simulink model "p4"  (R2020b)
settings: Solver=VariableStepAuto  StartTime=0.0  StopTime=10.0  RelTol=1e-3
model workspace (MAT data in the model file):
  a = 0.5
  b = 0.25
  x = 0.4
libraries: simulink x1
settings Model: OrderedModelArguments=off  Creator=DELL  LastModifiedBy=DELL

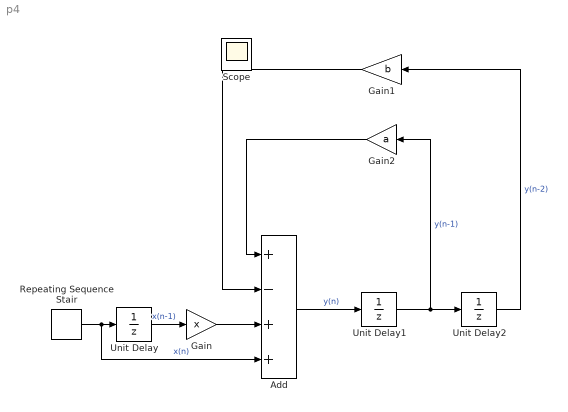
== system p4 ==
  Add : Sum  Inputs=+-++
  Gain : Gain  Gain=x
  Gain1 : Gain  Gain=b
  Gain2 : Gain  Gain=a
  Repeating Sequence Stair : simulink/Sources/Repeating Sequence Stair  OutValues=[3 1 4 2 1].'  tsamp=-1  OutMin=[]  OutMax=[]  OutDataTypeStr=double  OutputDataTypeScalingMode=double  OutDataType=fixdt(0,8)  ConRadixGroup=Best Precision: Vector-wise  OutScaling=2^-12
  Unit Delay : UnitDelay  SampleTime=-1  HasFrameUpgradeWarning=on
  Unit Delay1 : UnitDelay  SampleTime=-1  HasFrameUpgradeWarning=on
  Unit Delay2 : UnitDelay  SampleTime=-1  HasFrameUpgradeWarning=on
  Scope : Scope
  wires:
  Gain1/1 -> Add/2
  Add/1 -> Unit Delay1/1  "y(n)"
  Gain2/1 -> Add/1
  Unit Delay1/1 -> Gain2/1, Unit Delay2/1  "y(n-1)"
  Unit Delay2/1 -> Gain1/1  "y(n-2)"
  Gain/1 -> Add/3
  Unit Delay/1 -> Gain/1  "x(n-1)"
  Repeating Sequence Stair/1 -> Add/4, Unit Delay/1  "x(n)"
